simulink model "Series_RLC"  (R2022a)
settings: Solver=VariableStepAuto  StartTime=0.0  StopTime=5e-3  RelTol=1e-3
model workspace (MAT data in the model file):
  I_L_Init = 0
  V_C_Init = 0
undefined symbols (not defined in the file): C, I_L_init, L, R, V_C_init
settings Model: Creator=hitma  LastModifiedBy=hitma

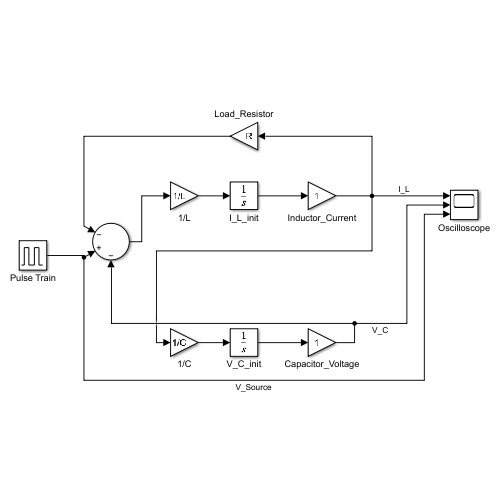
[thumbnail: Simulink's stored preview of the top-level diagram]
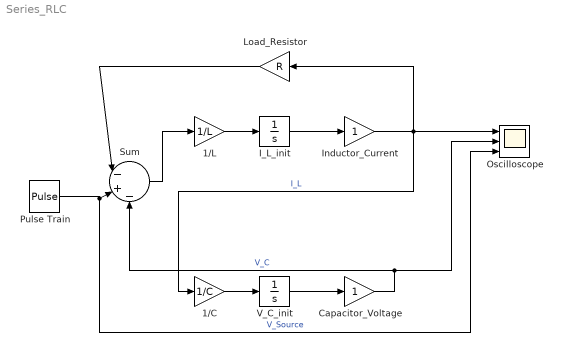
== system Series_RLC ==
  1/C : Gain  Gain=1/C
  1/L : Gain  Gain=1/L
  Capacitor_Voltage : Gain
  I_L_init : Integrator  InitialCondition=I_L_init
  Inductor_Current : Gain
  Load_Resistor : Gain  Gain=R
  Oscilloscope : Scope  NumInputPorts=3
  Pulse Train : DiscretePulseGenerator  PulseType=Time based  Amplitude=10  Period=1e-6  PulseWidth=90
  Sum : Sum  Inputs=|-+-
  V_C_init : Integrator  InitialCondition=V_C_init
  wires:
  1/L/1 -> I_L_init/1
  1/C/1 -> V_C_init/1
  Sum/1 -> 1/L/1
  Load_Resistor/1 -> Sum/1
  I_L_init/1 -> Inductor_Current/1
  V_C_init/1 -> Capacitor_Voltage/1
  Pulse Train/1 -> Oscilloscope/3, Sum/2  "V_Source"
  Inductor_Current/1 -> Load_Resistor/1, Oscilloscope/1, 1/C/1  "I_L"
  Capacitor_Voltage/1 -> Sum/3, Oscilloscope/2  "V_C"
